simulink model "yarpRead"  (Simulink 7.9)
settings: Solver=ode45  StartTime=0.0  StopTime=inf  RelTol=1e-3
settings Model: Creator=iron  LastModifiedBy=jorhabib
settings DebuggingCC: FcnCallInpInsideContextMsg=Use local settings
settings GRTTargetCC: CombineOutputUpdateFcns=off  GRTInterface=on

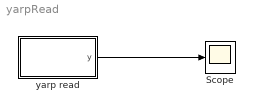
== system yarpRead ==
  Scope : Scope
      settings: YMin=-1.5e-05  YMax=5e-06
  yarp read : Subsystem  mask{port_name='/icub/left_arm/state:o', n=5}
      mask prompts: port_name "Specify port name starting with "/" e.g. '/port/input:i'"; n "Number of inputs"
  wires:
  yarp read/1(" y") -> Scope/1

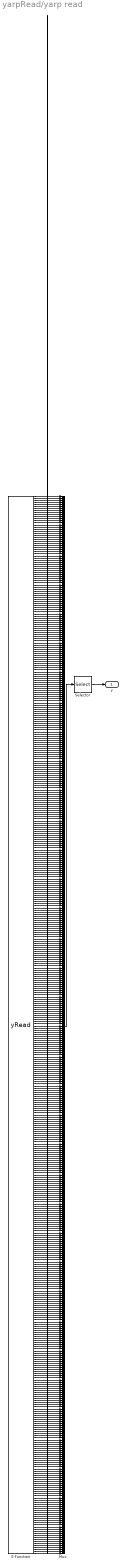
== system yarpRead/yarp read ==
  Mux : Mux  Inputs=512
  S-Function : S-Function  FunctionName=yRead  Parameters=port_name  EnableBusSupport=off
  Selector : Selector  InputPortWidth=512  IndexOptions=Index vector (dialog)  Indices=[1:n]  OutputSizes=1
  " y" : Outport
  wires:
  S-Function/1 -> Mux/1
  S-Function/2 -> Mux/2
  S-Function/3 -> Mux/3
  S-Function/4 -> Mux/4
  S-Function/5 -> Mux/5
  S-Function/6 -> Mux/6
  S-Function/7 -> Mux/7
  S-Function/8 -> Mux/8
  S-Function/9 -> Mux/9
  S-Function/10 -> Mux/10
  S-Function/11 -> Mux/11
  S-Function/12 -> Mux/12
  S-Function/13 -> Mux/13
  S-Function/14 -> Mux/14
  S-Function/15 -> Mux/15
  S-Function/16 -> Mux/16
  S-Function/17 -> Mux/17
  S-Function/18 -> Mux/18
  S-Function/19 -> Mux/19
  S-Function/20 -> Mux/20
  S-Function/21 -> Mux/21
  S-Function/22 -> Mux/22
  S-Function/23 -> Mux/23
  S-Function/24 -> Mux/24
  S-Function/25 -> Mux/25
  S-Function/26 -> Mux/26
  S-Function/27 -> Mux/27
  S-Function/28 -> Mux/28
  S-Function/29 -> Mux/29
  S-Function/30 -> Mux/30
  S-Function/31 -> Mux/31
  S-Function/32 -> Mux/32
  S-Function/33 -> Mux/33
  S-Function/34 -> Mux/34
  S-Function/35 -> Mux/35
  S-Function/36 -> Mux/36
  S-Function/37 -> Mux/37
  S-Function/38 -> Mux/38
  S-Function/39 -> Mux/39
  S-Function/40 -> Mux/40
  S-Function/41 -> Mux/41
  S-Function/42 -> Mux/42
  S-Function/43 -> Mux/43
  S-Function/44 -> Mux/44
  S-Function/45 -> Mux/45
  S-Function/46 -> Mux/46
  S-Function/47 -> Mux/47
  S-Function/48 -> Mux/48
  S-Function/49 -> Mux/49
  S-Function/50 -> Mux/50
  S-Function/51 -> Mux/51
  S-Function/52 -> Mux/52
  S-Function/53 -> Mux/53
  S-Function/54 -> Mux/54
  S-Function/55 -> Mux/55
  S-Function/56 -> Mux/56
  S-Function/57 -> Mux/57
  S-Function/58 -> Mux/58
  S-Function/59 -> Mux/59
  S-Function/60 -> Mux/60
  S-Function/61 -> Mux/61
  S-Function/62 -> Mux/62
  S-Function/63 -> Mux/63
  S-Function/64 -> Mux/64
  S-Function/65 -> Mux/65
  S-Function/66 -> Mux/66
  S-Function/67 -> Mux/67
  S-Function/68 -> Mux/68
  S-Function/69 -> Mux/69
  S-Function/70 -> Mux/70
  S-Function/71 -> Mux/71
  S-Function/72 -> Mux/72
  S-Function/73 -> Mux/73
  S-Function/74 -> Mux/74
  S-Function/75 -> Mux/75
  S-Function/76 -> Mux/76
  S-Function/77 -> Mux/77
  S-Function/78 -> Mux/78
  S-Function/79 -> Mux/79
  S-Function/80 -> Mux/80
  S-Function/81 -> Mux/81
  S-Function/82 -> Mux/82
  S-Function/83 -> Mux/83
  S-Function/84 -> Mux/84
  S-Function/85 -> Mux/85
  S-Function/86 -> Mux/86
  S-Function/87 -> Mux/87
  S-Function/88 -> Mux/88
  S-Function/89 -> Mux/89
  S-Function/90 -> Mux/90
  S-Function/91 -> Mux/91
  S-Function/92 -> Mux/92
  S-Function/93 -> Mux/93
  S-Function/94 -> Mux/94
  S-Function/95 -> Mux/95
  S-Function/96 -> Mux/96
  S-Function/97 -> Mux/97
  S-Function/98 -> Mux/98
  S-Function/99 -> Mux/99
  S-Function/100 -> Mux/100
  S-Function/101 -> Mux/101
  S-Function/102 -> Mux/102
  S-Function/103 -> Mux/103
  S-Function/104 -> Mux/104
  S-Function/105 -> Mux/105
  S-Function/106 -> Mux/106
  S-Function/107 -> Mux/107
  S-Function/108 -> Mux/108
  S-Function/109 -> Mux/109
  S-Function/110 -> Mux/110
  S-Function/111 -> Mux/111
  S-Function/112 -> Mux/112
  S-Function/113 -> Mux/113
  S-Function/114 -> Mux/114
  S-Function/115 -> Mux/115
  S-Function/116 -> Mux/116
  S-Function/117 -> Mux/117
  S-Function/118 -> Mux/118
  S-Function/119 -> Mux/119
  S-Function/120 -> Mux/120
  S-Function/121 -> Mux/121
  S-Function/122 -> Mux/122
  S-Function/123 -> Mux/123
  S-Function/124 -> Mux/124
  S-Function/125 -> Mux/125
  S-Function/126 -> Mux/126
  S-Function/127 -> Mux/127
  S-Function/128 -> Mux/128
  S-Function/129 -> Mux/129
  S-Function/130 -> Mux/130
  S-Function/131 -> Mux/131
  S-Function/132 -> Mux/132
  S-Function/133 -> Mux/133
  S-Function/134 -> Mux/134
  S-Function/135 -> Mux/135
  S-Function/136 -> Mux/136
  S-Function/137 -> Mux/137
  S-Function/138 -> Mux/138
  S-Function/139 -> Mux/139
  S-Function/140 -> Mux/140
  S-Function/141 -> Mux/141
  S-Function/142 -> Mux/142
  S-Function/143 -> Mux/143
  S-Function/144 -> Mux/144
  S-Function/145 -> Mux/145
  S-Function/146 -> Mux/146
  S-Function/147 -> Mux/147
  S-Function/148 -> Mux/148
  S-Function/149 -> Mux/149
  S-Function/150 -> Mux/150
  S-Function/151 -> Mux/151
  S-Function/152 -> Mux/152
  S-Function/153 -> Mux/153
  S-Function/154 -> Mux/154
  S-Function/155 -> Mux/155
  S-Function/156 -> Mux/156
  S-Function/157 -> Mux/157
  S-Function/158 -> Mux/158
  S-Function/159 -> Mux/159
  S-Function/160 -> Mux/160
  S-Function/161 -> Mux/161
  S-Function/162 -> Mux/162
  S-Function/163 -> Mux/163
  S-Function/164 -> Mux/164
  S-Function/165 -> Mux/165
  S-Function/166 -> Mux/166
  S-Function/167 -> Mux/167
  S-Function/168 -> Mux/168
  S-Function/169 -> Mux/169
  S-Function/170 -> Mux/170
  S-Function/171 -> Mux/171
  S-Function/172 -> Mux/172
  S-Function/173 -> Mux/173
  S-Function/174 -> Mux/174
  S-Function/175 -> Mux/175
  S-Function/176 -> Mux/176
  S-Function/177 -> Mux/177
  S-Function/178 -> Mux/178
  S-Function/179 -> Mux/179
  S-Function/180 -> Mux/180
  S-Function/181 -> Mux/181
  S-Function/182 -> Mux/182
  S-Function/183 -> Mux/183
  S-Function/184 -> Mux/184
  S-Function/185 -> Mux/185
  S-Function/186 -> Mux/186
  S-Function/187 -> Mux/187
  S-Function/188 -> Mux/188
  S-Function/189 -> Mux/189
  S-Function/190 -> Mux/190
  S-Function/191 -> Mux/191
  S-Function/192 -> Mux/192
  S-Function/193 -> Mux/193
  S-Function/194 -> Mux/194
  S-Function/195 -> Mux/195
  S-Function/196 -> Mux/196
  S-Function/197 -> Mux/197
  S-Function/198 -> Mux/198
  S-Function/199 -> Mux/199
  S-Function/200 -> Mux/200
  S-Function/201 -> Mux/201
  S-Function/202 -> Mux/202
  S-Function/203 -> Mux/203
  S-Function/204 -> Mux/204
  S-Function/205 -> Mux/205
  S-Function/206 -> Mux/206
  S-Function/207 -> Mux/207
  S-Function/208 -> Mux/208
  S-Function/209 -> Mux/209
  S-Function/210 -> Mux/210
  S-Function/211 -> Mux/211
  S-Function/212 -> Mux/212
  S-Function/213 -> Mux/213
  S-Function/214 -> Mux/214
  S-Function/215 -> Mux/215
  S-Function/216 -> Mux/216
  S-Function/217 -> Mux/217
  S-Function/218 -> Mux/218
  S-Function/219 -> Mux/219
  S-Function/220 -> Mux/220
  S-Function/221 -> Mux/221
  S-Function/222 -> Mux/222
  S-Function/223 -> Mux/223
  S-Function/224 -> Mux/224
  S-Function/225 -> Mux/225
  S-Function/226 -> Mux/226
  S-Function/227 -> Mux/227
  S-Function/228 -> Mux/228
  S-Function/229 -> Mux/229
  S-Function/230 -> Mux/230
  S-Function/231 -> Mux/231
  S-Function/232 -> Mux/232
  S-Function/233 -> Mux/233
  S-Function/234 -> Mux/234
  S-Function/235 -> Mux/235
  S-Function/236 -> Mux/236
  S-Function/237 -> Mux/237
  S-Function/238 -> Mux/238
  S-Function/239 -> Mux/239
  S-Function/240 -> Mux/240
  S-Function/241 -> Mux/241
  S-Function/242 -> Mux/242
  S-Function/243 -> Mux/243
  S-Function/244 -> Mux/244
  S-Function/245 -> Mux/245
  S-Function/246 -> Mux/246
  S-Function/247 -> Mux/247
  S-Function/248 -> Mux/248
  S-Function/249 -> Mux/249
  S-Function/250 -> Mux/250
  S-Function/251 -> Mux/251
  S-Function/252 -> Mux/252
  S-Function/253 -> Mux/253
  S-Function/254 -> Mux/254
  S-Function/255 -> Mux/255
  S-Function/256 -> Mux/256
  S-Function/257 -> Mux/257
  S-Function/258 -> Mux/258
  S-Function/259 -> Mux/259
  S-Function/260 -> Mux/260
  S-Function/261 -> Mux/261
  S-Function/262 -> Mux/262
  S-Function/263 -> Mux/263
  S-Function/264 -> Mux/264
  S-Function/265 -> Mux/265
  S-Function/266 -> Mux/266
  S-Function/267 -> Mux/267
  S-Function/268 -> Mux/268
  S-Function/269 -> Mux/269
  S-Function/270 -> Mux/270
  S-Function/271 -> Mux/271
  S-Function/272 -> Mux/272
  S-Function/273 -> Mux/273
  S-Function/274 -> Mux/274
  S-Function/275 -> Mux/275
  S-Function/276 -> Mux/276
  S-Function/277 -> Mux/277
  S-Function/278 -> Mux/278
  S-Function/279 -> Mux/279
  S-Function/280 -> Mux/280
  S-Function/281 -> Mux/281
  S-Function/282 -> Mux/282
  S-Function/283 -> Mux/283
  S-Function/284 -> Mux/284
  S-Function/285 -> Mux/285
  S-Function/286 -> Mux/286
  S-Function/287 -> Mux/287
  S-Function/288 -> Mux/288
  S-Function/289 -> Mux/289
  S-Function/290 -> Mux/290
  S-Function/291 -> Mux/291
  S-Function/292 -> Mux/292
  S-Function/293 -> Mux/293
  S-Function/294 -> Mux/294
  S-Function/295 -> Mux/295
  S-Function/296 -> Mux/296
  S-Function/297 -> Mux/297
  S-Function/298 -> Mux/298
  S-Function/299 -> Mux/299
  S-Function/300 -> Mux/300
  S-Function/301 -> Mux/301
  S-Function/302 -> Mux/302
  S-Function/303 -> Mux/303
  S-Function/304 -> Mux/304
  S-Function/305 -> Mux/305
  S-Function/306 -> Mux/306
  S-Function/307 -> Mux/307
  S-Function/308 -> Mux/308
  S-Function/309 -> Mux/309
  S-Function/310 -> Mux/310
  S-Function/311 -> Mux/311
  S-Function/312 -> Mux/312
  S-Function/313 -> Mux/313
  S-Function/314 -> Mux/314
  S-Function/315 -> Mux/315
  S-Function/316 -> Mux/316
  S-Function/317 -> Mux/317
  S-Function/318 -> Mux/318
  S-Function/319 -> Mux/319
  S-Function/320 -> Mux/320
  S-Function/321 -> Mux/321
  S-Function/322 -> Mux/322
  S-Function/323 -> Mux/323
  S-Function/324 -> Mux/324
  S-Function/325 -> Mux/325
  S-Function/326 -> Mux/326
  S-Function/327 -> Mux/327
  S-Function/328 -> Mux/328
  S-Function/329 -> Mux/329
  S-Function/330 -> Mux/330
  S-Function/331 -> Mux/331
  S-Function/332 -> Mux/332
  S-Function/333 -> Mux/333
  S-Function/334 -> Mux/334
  S-Function/335 -> Mux/335
  S-Function/336 -> Mux/336
  S-Function/337 -> Mux/337
  S-Function/338 -> Mux/338
  S-Function/339 -> Mux/339
  S-Function/340 -> Mux/340
  S-Function/341 -> Mux/341
  S-Function/342 -> Mux/342
  S-Function/343 -> Mux/343
  S-Function/344 -> Mux/344
  S-Function/345 -> Mux/345
  S-Function/346 -> Mux/346
  S-Function/347 -> Mux/347
  S-Function/348 -> Mux/348
  S-Function/349 -> Mux/349
  S-Function/350 -> Mux/350
  S-Function/351 -> Mux/351
  S-Function/352 -> Mux/352
  S-Function/353 -> Mux/353
  S-Function/354 -> Mux/354
  S-Function/355 -> Mux/355
  S-Function/356 -> Mux/356
  S-Function/357 -> Mux/357
  S-Function/358 -> Mux/358
  S-Function/359 -> Mux/359
  S-Function/360 -> Mux/360
  S-Function/361 -> Mux/361
  S-Function/362 -> Mux/362
  S-Function/363 -> Mux/363
  S-Function/364 -> Mux/364
  S-Function/365 -> Mux/365
  S-Function/366 -> Mux/366
  S-Function/367 -> Mux/367
  S-Function/368 -> Mux/368
  S-Function/369 -> Mux/369
  S-Function/370 -> Mux/370
  S-Function/371 -> Mux/371
  S-Function/372 -> Mux/372
  S-Function/373 -> Mux/373
  S-Function/374 -> Mux/374
  S-Function/375 -> Mux/375
  S-Function/376 -> Mux/376
  S-Function/377 -> Mux/377
  S-Function/378 -> Mux/378
  S-Function/379 -> Mux/379
  S-Function/380 -> Mux/380
  S-Function/381 -> Mux/381
  S-Function/382 -> Mux/382
  S-Function/383 -> Mux/383
  S-Function/384 -> Mux/384
  S-Function/385 -> Mux/385
  S-Function/386 -> Mux/386
  S-Function/387 -> Mux/387
  S-Function/388 -> Mux/388
  S-Function/389 -> Mux/389
  S-Function/390 -> Mux/390
  S-Function/391 -> Mux/391
  S-Function/392 -> Mux/392
  S-Function/393 -> Mux/393
  S-Function/394 -> Mux/394
  S-Function/395 -> Mux/395
  S-Function/396 -> Mux/396
  S-Function/397 -> Mux/397
  S-Function/398 -> Mux/398
  S-Function/399 -> Mux/399
  S-Function/400 -> Mux/400
  S-Function/401 -> Mux/401
  S-Function/402 -> Mux/402
  S-Function/403 -> Mux/403
  S-Function/404 -> Mux/404
  S-Function/405 -> Mux/405
  S-Function/406 -> Mux/406
  S-Function/407 -> Mux/407
  S-Function/408 -> Mux/408
  S-Function/409 -> Mux/409
  S-Function/410 -> Mux/410
  S-Function/411 -> Mux/411
  S-Function/412 -> Mux/412
  S-Function/413 -> Mux/413
  S-Function/414 -> Mux/414
  S-Function/415 -> Mux/415
  S-Function/416 -> Mux/416
  S-Function/417 -> Mux/417
  S-Function/418 -> Mux/418
  S-Function/419 -> Mux/419
  S-Function/420 -> Mux/420
  S-Function/421 -> Mux/421
  S-Function/422 -> Mux/422
  S-Function/423 -> Mux/423
  S-Function/424 -> Mux/424
  S-Function/425 -> Mux/425
  S-Function/426 -> Mux/426
  S-Function/427 -> Mux/427
  S-Function/428 -> Mux/428
  S-Function/429 -> Mux/429
  S-Function/430 -> Mux/430
  S-Function/431 -> Mux/431
  S-Function/432 -> Mux/432
  S-Function/433 -> Mux/433
  S-Function/434 -> Mux/434
  S-Function/435 -> Mux/435
  S-Function/436 -> Mux/436
  S-Function/437 -> Mux/437
  S-Function/438 -> Mux/438
  S-Function/439 -> Mux/439
  S-Function/440 -> Mux/440
  S-Function/441 -> Mux/441
  S-Function/442 -> Mux/442
  S-Function/443 -> Mux/443
  S-Function/444 -> Mux/444
  S-Function/445 -> Mux/445
  S-Function/446 -> Mux/446
  S-Function/447 -> Mux/447
  S-Function/448 -> Mux/448
  S-Function/449 -> Mux/449
  S-Function/450 -> Mux/450
  S-Function/451 -> Mux/451
  S-Function/452 -> Mux/452
  S-Function/453 -> Mux/453
  S-Function/454 -> Mux/454
  S-Function/455 -> Mux/455
  S-Function/456 -> Mux/456
  S-Function/457 -> Mux/457
  S-Function/458 -> Mux/458
  S-Function/459 -> Mux/459
  S-Function/460 -> Mux/460
  S-Function/461 -> Mux/461
  S-Function/462 -> Mux/462
  S-Function/463 -> Mux/463
  S-Function/464 -> Mux/464
  S-Function/465 -> Mux/465
  S-Function/466 -> Mux/466
  S-Function/467 -> Mux/467
  S-Function/468 -> Mux/468
  S-Function/469 -> Mux/469
  S-Function/470 -> Mux/470
  S-Function/471 -> Mux/471
  S-Function/472 -> Mux/472
  S-Function/473 -> Mux/473
  S-Function/474 -> Mux/474
  S-Function/475 -> Mux/475
  S-Function/476 -> Mux/476
  S-Function/477 -> Mux/477
  S-Function/478 -> Mux/478
  S-Function/479 -> Mux/479
  S-Function/480 -> Mux/480
  S-Function/481 -> Mux/481
  S-Function/482 -> Mux/482
  S-Function/483 -> Mux/483
  S-Function/484 -> Mux/484
  S-Function/485 -> Mux/485
  S-Function/486 -> Mux/486
  S-Function/487 -> Mux/487
  S-Function/488 -> Mux/488
  S-Function/489 -> Mux/489
  S-Function/490 -> Mux/490
  S-Function/491 -> Mux/491
  S-Function/492 -> Mux/492
  S-Function/493 -> Mux/493
  S-Function/494 -> Mux/494
  S-Function/495 -> Mux/495
  S-Function/496 -> Mux/496
  S-Function/497 -> Mux/497
  S-Function/498 -> Mux/498
  S-Function/499 -> Mux/499
  S-Function/500 -> Mux/500
  S-Function/501 -> Mux/501
  S-Function/502 -> Mux/502
  S-Function/503 -> Mux/503
  S-Function/504 -> Mux/504
  S-Function/505 -> Mux/505
  S-Function/506 -> Mux/506
  S-Function/507 -> Mux/507
  S-Function/508 -> Mux/508
  S-Function/509 -> Mux/509
  S-Function/510 -> Mux/510
  S-Function/511 -> Mux/511
  S-Function/512 -> Mux/512
  Mux/1 -> Selector/1
  Selector/1 -> " y"/1
